simulink model "LinearMPC_noConstraints"  (R2021b)
settings: Solver=FixedStepDiscrete  StartTime=0.0  StopTime=20.0  FixedStep=Ts  RelTol=1e-3  EnableMultiTasking=on
values from neighbouring files (symbols this model uses):
  A = sysd.A    [es_4.m]
  B = sysd.B    [es_4.m]
  C_states = eye(2)    [es_4.m]
  D_states = [0 0]'    [es_4.m]
  N = 5    [es_4.m]
  N2 = 100    [es_4.m]
  QMPC = Q_LQ    [es_4.m]
  QMPC2 = Q_LQ    [es_4.m]
  R = R_LQ    (= 1)    [es_4.m]
  sat_max = umax    (= 5)    [es_4.m]
  sat_min = umin    (= -5)    [es_4.m]
  sysd = c2d(sys,Ts)    [es_4.m]
  Ts = 0.1    [es_4.m]
  x0 = [0 10]'    [es_4.m]
  xref = [0 0]'    [es_4.m]
undefined symbols (not defined in the file or in its folder): mympc, Pr, Pr2
settings Model: Creator=Mirko  LastModifiedBy=Chiara
settings SolverCC: AlgebraicLoopSolver=TrustRegion
settings DataIOCC: LimitDataPoints=on  SaveFormat=Array  SignalLoggingSaveFormat=ModelDataLogs  ReturnWorkspaceOutputs=off
settings OptimizationCC: ExpressionDepthLimit=2147483647  LifeSpan=inf
settings DebuggingCC: UnderspecifiedInitializationDetection=Classic  MergeDetectMultiDrivingBlocksExec=none  SolverPrmCheckMsg=warning  FcnCallInpInsideContextMsg=warning  StateNameClashWarn=warning  SFUnexpectedBacktrackingDiag=warning  SFNoUnconditionalDefaultTransitionDiag=warning  SFExecutionAtInitializationDiag=none  SFMachineParentedDataDiag=warning  ArithmeticOperatorsInVariantConditions=warning
settings HardwareCC: ProdBitPerPointer=32  ProdBitPerSizeT=32  ProdBitPerPtrDiffT=32  ProdLargestAtomicFloat=None  ProdIntDivRoundTo=Undefined  ProdEndianess=Unspecified  ProdWordSize=32  ProdHWDeviceType=32-bit Generic
settings ModelReferenceCC: PropagateSignalLabelsOutOfModel=off
settings SFSimCC: SimUseLocalCustomCode=off  CustomCodeUndefinedFunction=UseInterfaceOnly
settings RTWCC: RTWUseLocalCustomCode=off
settings CodeAppCC: StateflowObjectComments=on
settings GRTTargetCC: TargetLangStandard=C89/C90 (ANSI)
settings ConfigComp: CovMetricSettings=dw  CovSaveCumulativeToWorkspaceVar=on  CovSaveSingleToWorkspaceVar=on  CovExternalEMLEnable=off  CovSFcnEnable=off

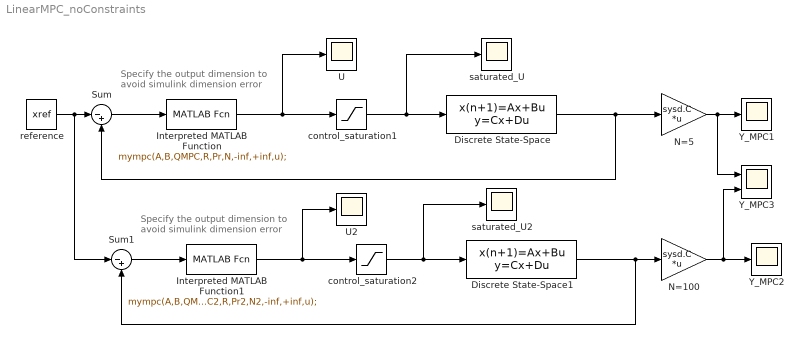
== system LinearMPC_noConstraints ==
  note: Specify the output dimension
      | to avoid simulink dimension error
  note: Specify the output dimension
      | to avoid simulink dimension error
  Discrete State-Space : DiscreteStateSpace  A=sysd.A  B=sysd.B  C=C_states  D=D_states  InitialCondition=x0  SampleTime=Ts
  Discrete State-Space1 : DiscreteStateSpace  A=sysd.A  B=sysd.B  C=C_states  D=D_states  InitialCondition=x0  SampleTime=Ts
  Interpreted MATLAB Function : MATLABFcn  MATLABFcn=mympc(A,B,QMPC,R,Pr,N,-inf,+inf,u);  OutputDimensions=1
  Interpreted MATLAB Function1 : MATLABFcn  MATLABFcn=mympc(A,B,QMPC2,R,Pr2,N2,-inf,+inf,u);  OutputDimensions=1
  N=100 : Gain  Gain=sysd.C  Multiplication=Matrix(K*u) (u vector)
  N=5 : Gain  Gain=sysd.C  Multiplication=Matrix(K*u) (u vector)
  Sum : Sum  Inputs=|-+
  Sum1 : Sum  Inputs=|-+
  U : Scope
  U2 : Scope
  Y_MPC1 : Scope
  Y_MPC2 : Scope
  Y_MPC3 : Scope  NumInputPorts=2
  control_saturation1 : Saturate  UpperLimit=sat_max  LowerLimit=sat_min
  control_saturation2 : Saturate  UpperLimit=sat_max  LowerLimit=sat_min
  reference : Constant  Value=xref
  saturated_U : Scope
  saturated_U2 : Scope
  wires:
  Discrete State-Space/1 -> Sum/2, N=5/1
  Sum/1 -> Interpreted MATLAB Function/1
  N=5/1 -> Y_MPC3/1, Y_MPC1/1
  Interpreted MATLAB Function/1 -> control_saturation1/1, U/1
  control_saturation1/1 -> saturated_U/1, Discrete State-Space/1
  Discrete State-Space1/1 -> Sum1/2, N=100/1
  reference/1 -> Sum1/1, Sum/1
  Interpreted MATLAB Function1/1 -> control_saturation2/1, U2/1
  Sum1/1 -> Interpreted MATLAB Function1/1
  control_saturation2/1 -> saturated_U2/1, Discrete State-Space1/1
  N=100/1 -> Y_MPC3/2, Y_MPC2/1
